simulink model "IEEE33BusTestSystemSimple"  (Simulink 10.3)
settings: Solver=FixedStepAuto  StartTime=0.0  StopTime=0.2  RelTol=1e-3
undefined symbols (not defined in the file): D1, Delta
libraries: spsThreePhaseVIMeasurementLib x43, spsThreePhaseSeriesRLCBranchLib x39, spsThreePhaseSeriesRLCLoadLib x34, simulink_extras x9, spsFrequencyPhasorLib x9, spsPowerPositiveSequenceLib x9, spsSequenceAnalyzerLib x9, spsThreePhaseParallelRLCLoadLib x3, spsSeriesRLCBranchLib x3, spsAC1AExcitationSystemLib x2, spsDieselMotorModel x2, spsSynchronousMachinepuStandardLib x2
(part 2 of 3)

== system IEEE33BusTestSystemSimple/Bus_18 ==
  Bus Load 18 : spsThreePhaseSeriesRLCLoadLib/Three-Phase Series RLC Load  LConnTagsString=A|B|C  Configuration=Y (grounded)  NominalVoltage=(12660)*0.91322  Vabc=[1e3 1e3 1e3]  Vabcp=[1e3 1e3 1e3]  NominalFrequency=50  UnbalancedPower=off  ActivePower=90e3  InductivePower=40e3  CapacitivePower=0  Pabc=[10e3 9e3 11e3]  QLabc=[100 90 110]  QCabc=[100 90 110]  Pabcp=[10e3 9e3 11e3]  QLabcp=[100 90 110]  QCabcp=[100 90 110]  Measurements=None  LoadType=constant PQ
  Bus_18 : spsThreePhaseVIMeasurementLib/Three-Phase V-I Measurement  VoltageMeasurement=phase-to-phase  SetLabelV=off  LabelV=Vabc  Vpu=off  VpuLL=off  CurrentMeasurement=yes  SetLabelI=off  LabelI=Iabc  Ipu=off  Pbase=100e6  Vbase=500e3  OutputType=Complex  PhasorSimulation=off  PSBequivalent=0
  VI Recorder21 : Subsystem
  InPhaseA : PMIOPort  Side=Left
  InPhaseB : PMIOPort  Port=2  Side=Left
  InPhaseC : PMIOPort  Port=3  Side=Left
  OutPhaseA : PMIOPort  Port=4  Side=Right
  OutPhaseB : PMIOPort  Port=5  Side=Right
  OutPhaseC : PMIOPort  Port=6  Side=Right
  wires:
  Bus_18/1 -> VI Recorder21/1(Vrec)
  Bus_18/2 -> VI Recorder21/2(Irec)
  connections:
  Bus Load 18/LConn1 -- OutPhaseA/RConn1 -- Bus_18/RConn1
  Bus_18/RConn2 -- OutPhaseB/RConn1 -- Bus Load 18/LConn2
  Bus_18/RConn3 -- OutPhaseC/RConn1 -- Bus Load 18/LConn3
  InPhaseA/RConn1 -- Bus_18/LConn1
  InPhaseB/RConn1 -- Bus_18/LConn2
  InPhaseC/RConn1 -- Bus_18/LConn3

== system IEEE33BusTestSystemSimple/Bus_19 ==
  Bus Load 19 : spsThreePhaseSeriesRLCLoadLib/Three-Phase Series RLC Load  LConnTagsString=A|B|C  Configuration=Y (grounded)  NominalVoltage=(12660)*0.996507  Vabc=[1e3 1e3 1e3]  Vabcp=[1e3 1e3 1e3]  NominalFrequency=50  UnbalancedPower=off  ActivePower=90e3  InductivePower=40e3  CapacitivePower=0  Pabc=[10e3 9e3 11e3]  QLabc=[100 90 110]  QCabc=[100 90 110]  Pabcp=[10e3 9e3 11e3]  QLabcp=[100 90 110]  QCabcp=[100 90 110]  Measurements=None  LoadType=constant PQ
  Bus_19 : spsThreePhaseVIMeasurementLib/Three-Phase V-I Measurement  VoltageMeasurement=phase-to-phase  SetLabelV=off  LabelV=Vabc  Vpu=off  VpuLL=off  CurrentMeasurement=yes  SetLabelI=off  LabelI=Iabc  Ipu=off  Pbase=100e6  Vbase=500e3  OutputType=Complex  PhasorSimulation=off  PSBequivalent=0
  VI Recorder : Subsystem
  InPhaseA : PMIOPort  Side=Left
  InPhaseB : PMIOPort  Port=2  Side=Left
  InPhaseC : PMIOPort  Port=3  Side=Left
  OutPhaseA : PMIOPort  Port=4  Side=Right
  OutPhaseB : PMIOPort  Port=5  Side=Right
  OutPhaseC : PMIOPort  Port=6  Side=Right
  wires:
  Bus_19/2 -> VI Recorder/2(Irec)
  Bus_19/1 -> VI Recorder/1(Vrec)
  connections:
  Bus Load 19/LConn1 -- OutPhaseA/RConn1 -- Bus_19/RConn1
  Bus_19/RConn2 -- OutPhaseB/RConn1 -- Bus Load 19/LConn2
  Bus Load 19/LConn3 -- OutPhaseC/RConn1 -- Bus_19/RConn3
  Bus_19/LConn1 -- InPhaseA/RConn1
  InPhaseB/RConn1 -- Bus_19/LConn2
  InPhaseC/RConn1 -- Bus_19/LConn3

== system IEEE33BusTestSystemSimple/Bus_2 ==
  Bus Load 2 : spsThreePhaseSeriesRLCLoadLib/Three-Phase Series RLC Load  LConnTagsString=A|B|C  Configuration=Y (grounded)  NominalVoltage=(12660)*0.997035  Vabc=[1e3 1e3 1e3]  Vabcp=[1e3 1e3 1e3]  NominalFrequency=50  UnbalancedPower=off  ActivePower=100e3  InductivePower=60e3  CapacitivePower=0  Pabc=[10e3 9e3 11e3]  QLabc=[100 90 110]  QCabc=[100 90 110]  Pabcp=[10e3 9e3 11e3]  QLabcp=[100 90 110]  QCabcp=[100 90 110]  Measurements=None  LoadType=constant PQ
  Bus_2 : spsThreePhaseVIMeasurementLib/Three-Phase V-I Measurement  VoltageMeasurement=phase-to-phase  SetLabelV=off  LabelV=Vabc  Vpu=off  VpuLL=off  CurrentMeasurement=yes  SetLabelI=off  LabelI=Iabc  Ipu=off  Pbase=100e6  Vbase=500e3  OutputType=Complex  PhasorSimulation=off  PSBequivalent=0
  VI Recorder5 : Subsystem
  InPhaseA : PMIOPort  Side=Left
  InPhaseB : PMIOPort  Port=2  Side=Left
  InPhaseC : PMIOPort  Port=3  Side=Left
  OutPhaseA1 : PMIOPort  Port=4  Side=Right
  OutPhaseB1 : PMIOPort  Port=5  Side=Right
  OutPhaseC1 : PMIOPort  Port=6  Side=Right
  OutPhaseA : PMIOPort  Port=7  Side=Right
  OutPhaseB : PMIOPort  Port=8  Side=Right
  OutPhaseC : PMIOPort  Port=9  Side=Right
  wires:
  Bus_2/2 -> VI Recorder5/2(Irec)
  Bus_2/1 -> VI Recorder5/1(Vrec)
  connections:
  InPhaseC/RConn1 -- Bus_2/LConn3
  InPhaseB/RConn1 -- Bus_2/LConn2
  InPhaseA/RConn1 -- Bus_2/LConn1
  Bus Load 2/LConn1 -- OutPhaseA1/RConn1 -- OutPhaseA/RConn1 -- Bus_2/RConn1
  Bus Load 2/LConn2 -- OutPhaseB1/RConn1 -- OutPhaseB/RConn1 -- Bus_2/RConn2
  Bus Load 2/LConn3 -- OutPhaseC1/RConn1 -- OutPhaseC/RConn1 -- Bus_2/RConn3

== system IEEE33BusTestSystemSimple/Bus_20 ==
  Bus Load 20 : spsThreePhaseSeriesRLCLoadLib/Three-Phase Series RLC Load  LConnTagsString=A|B|C  Configuration=Y (grounded)  NominalVoltage=(12660)*0.992929  Vabc=[1e3 1e3 1e3]  Vabcp=[1e3 1e3 1e3]  NominalFrequency=50  UnbalancedPower=off  ActivePower=90e3  InductivePower=40e3  CapacitivePower=0  Pabc=[10e3 9e3 11e3]  QLabc=[100 90 110]  QCabc=[100 90 110]  Pabcp=[10e3 9e3 11e3]  QLabcp=[100 90 110]  QCabcp=[100 90 110]  Measurements=None  LoadType=constant PQ
  Bus_20 : spsThreePhaseVIMeasurementLib/Three-Phase V-I Measurement  VoltageMeasurement=phase-to-phase  SetLabelV=off  LabelV=Vabc  Vpu=off  VpuLL=off  CurrentMeasurement=yes  SetLabelI=off  LabelI=Iabc  Ipu=off  Pbase=100e6  Vbase=500e3  OutputType=Complex  PhasorSimulation=off  PSBequivalent=0
  VI Recorder1 : Subsystem
  InPhaseA : PMIOPort  Side=Left
  InPhaseB : PMIOPort  Port=2  Side=Left
  InPhaseC : PMIOPort  Port=3  Side=Left
  OutPhaseA : PMIOPort  Port=4  Side=Right
  OutPhaseB : PMIOPort  Port=5  Side=Right
  OutPhaseC : PMIOPort  Port=6  Side=Right
  wires:
  Bus_20/1 -> VI Recorder1/1(Vrec)
  Bus_20/2 -> VI Recorder1/2(Irec)
  connections:
  Bus Load 20/LConn1 -- OutPhaseA/RConn1 -- Bus_20/RConn1
  Bus_20/RConn2 -- OutPhaseB/RConn1 -- Bus Load 20/LConn2
  Bus Load 20/LConn3 -- OutPhaseC/RConn1 -- Bus_20/RConn3
  InPhaseA/RConn1 -- Bus_20/LConn1
  InPhaseB/RConn1 -- Bus_20/LConn2
  InPhaseC/RConn1 -- Bus_20/LConn3

== system IEEE33BusTestSystemSimple/Bus_21 ==
  Bus Load 21 : spsThreePhaseSeriesRLCLoadLib/Three-Phase Series RLC Load  LConnTagsString=A|B|C  Configuration=Y (grounded)  NominalVoltage=(12660)*0.992224  Vabc=[1e3 1e3 1e3]  Vabcp=[1e3 1e3 1e3]  NominalFrequency=50  UnbalancedPower=off  ActivePower=90e3  InductivePower=40e3  CapacitivePower=0  Pabc=[10e3 9e3 11e3]  QLabc=[100 90 110]  QCabc=[100 90 110]  Pabcp=[10e3 9e3 11e3]  QLabcp=[100 90 110]  QCabcp=[100 90 110]  Measurements=None  LoadType=constant PQ
  Bus_21 : spsThreePhaseVIMeasurementLib/Three-Phase V-I Measurement  VoltageMeasurement=phase-to-phase  SetLabelV=off  LabelV=Vabc  Vpu=off  VpuLL=off  CurrentMeasurement=yes  SetLabelI=off  LabelI=Iabc  Ipu=off  Pbase=100e6  Vbase=500e3  OutputType=Complex  PhasorSimulation=off  PSBequivalent=0
  VI Recorder2 : Subsystem
  InPhaseA : PMIOPort  Side=Left
  InPhaseB : PMIOPort  Port=2  Side=Left
  InPhaseC : PMIOPort  Port=3  Side=Left
  OutPhaseA : PMIOPort  Port=4  Side=Right
  OutPhaseB : PMIOPort  Port=5  Side=Right
  OutPhaseC : PMIOPort  Port=6  Side=Right
  OutPhaseA1 : PMIOPort  Port=7  Side=Right
  OutPhaseB1 : PMIOPort  Port=8  Side=Right
  OutPhaseC1 : PMIOPort  Port=9  Side=Right
  wires:
  Bus_21/2 -> VI Recorder2/2(Irec)
  Bus_21/1 -> VI Recorder2/1(Vrec)
  connections:
  Bus_21/RConn1 -- OutPhaseA/RConn1 -- OutPhaseA1/RConn1 -- Bus Load 21/LConn1
  Bus_21/RConn2 -- OutPhaseB/RConn1 -- OutPhaseB1/RConn1 -- Bus Load 21/LConn2
  InPhaseA/RConn1 -- Bus_21/LConn1
  Bus_21/LConn2 -- InPhaseB/RConn1
  InPhaseC/RConn1 -- Bus_21/LConn3
  Bus Load 21/LConn3 -- OutPhaseC/RConn1 -- OutPhaseC1/RConn1 -- Bus_21/RConn3

== system IEEE33BusTestSystemSimple/Bus_22 ==
  Bus Load 22 : spsThreePhaseSeriesRLCLoadLib/Three-Phase Series RLC Load  LConnTagsString=A|B|C  Configuration=Y (grounded)  NominalVoltage=(12660)*0.991587  Vabc=[1e3 1e3 1e3]  Vabcp=[1e3 1e3 1e3]  NominalFrequency=50  UnbalancedPower=off  ActivePower=90e3  InductivePower=40e3  CapacitivePower=0  Pabc=[10e3 9e3 11e3]  QLabc=[100 90 110]  QCabc=[100 90 110]  Pabcp=[10e3 9e3 11e3]  QLabcp=[100 90 110]  QCabcp=[100 90 110]  Measurements=None  LoadType=constant PQ
  Bus_22 : spsThreePhaseVIMeasurementLib/Three-Phase V-I Measurement  VoltageMeasurement=phase-to-phase  SetLabelV=off  LabelV=Vabc  Vpu=off  VpuLL=off  CurrentMeasurement=yes  SetLabelI=off  LabelI=Iabc  Ipu=off  Pbase=100e6  Vbase=500e3  OutputType=Complex  PhasorSimulation=off  PSBequivalent=0
  VI Recorder3 : Subsystem
  InPhaseA : PMIOPort  Side=Left
  InPhaseB : PMIOPort  Port=2  Side=Left
  InPhaseC : PMIOPort  Port=3  Side=Left
  OutPhaseA : PMIOPort  Port=4  Side=Right
  OutPhaseB : PMIOPort  Port=5  Side=Right
  OutPhaseC : PMIOPort  Port=6  Side=Right
  wires:
  Bus_22/2 -> VI Recorder3/2(Irec)
  Bus_22/1 -> VI Recorder3/1(Vrec)
  connections:
  Bus_22/RConn2 -- OutPhaseB/RConn1 -- Bus Load 22/LConn2
  Bus Load 22/LConn3 -- OutPhaseC/RConn1 -- Bus_22/RConn3
  Bus_22/RConn1 -- OutPhaseA/RConn1 -- Bus Load 22/LConn1
  InPhaseA/RConn1 -- Bus_22/LConn1
  InPhaseB/RConn1 -- Bus_22/LConn2
  InPhaseC/RConn1 -- Bus_22/LConn3

== system IEEE33BusTestSystemSimple/Bus_23 ==
  Bus Load 23 : spsThreePhaseSeriesRLCLoadLib/Three-Phase Series RLC Load  LConnTagsString=A|B|C  Configuration=Y (grounded)  NominalVoltage=(12660)*0.97937  Vabc=[1e3 1e3 1e3]  Vabcp=[1e3 1e3 1e3]  NominalFrequency=50  UnbalancedPower=off  ActivePower=90e3  InductivePower=50e3  CapacitivePower=0  Pabc=[10e3 9e3 11e3]  QLabc=[100 90 110]  QCabc=[100 90 110]  Pabcp=[10e3 9e3 11e3]  QLabcp=[100 90 110]  QCabcp=[100 90 110]  Measurements=None  LoadType=constant PQ
  Bus_23 : spsThreePhaseVIMeasurementLib/Three-Phase V-I Measurement  VoltageMeasurement=phase-to-phase  SetLabelV=off  LabelV=Vabc  Vpu=off  VpuLL=off  CurrentMeasurement=yes  SetLabelI=off  LabelI=Iabc  Ipu=off  Pbase=100e6  Vbase=500e3  OutputType=Complex  PhasorSimulation=off  PSBequivalent=0
  VI Recorder32 : Subsystem
  InPhaseA : PMIOPort  Side=Left
  InPhaseB : PMIOPort  Port=2  Side=Left
  InPhaseC : PMIOPort  Port=3  Side=Left
  OutPhaseA : PMIOPort  Port=4  Side=Right
  OutPhaseB : PMIOPort  Port=5  Side=Right
  OutPhaseC : PMIOPort  Port=6  Side=Right
  wires:
  Bus_23/2 -> VI Recorder32/2(Irec)
  Bus_23/1 -> VI Recorder32/1(Vrec)
  connections:
  Bus Load 23/LConn1 -- OutPhaseA/RConn1 -- Bus_23/RConn1
  Bus_23/RConn2 -- OutPhaseB/RConn1 -- Bus Load 23/LConn2
  Bus_23/RConn3 -- OutPhaseC/RConn1 -- Bus Load 23/LConn3
  InPhaseA/RConn1 -- Bus_23/LConn1
  InPhaseB/RConn1 -- Bus_23/LConn2
  InPhaseC/RConn1 -- Bus_23/LConn3

== system IEEE33BusTestSystemSimple/Bus_24 ==
  Bus Load 24 : spsThreePhaseSeriesRLCLoadLib/Three-Phase Series RLC Load  LConnTagsString=A|B|C  Configuration=Y (grounded)  NominalVoltage=(12660)*0.9727  Vabc=[1e3 1e3 1e3]  Vabcp=[1e3 1e3 1e3]  NominalFrequency=50  UnbalancedPower=off  ActivePower=420e3  InductivePower=200e3  CapacitivePower=0  Pabc=[10e3 9e3 11e3]  QLabc=[100 90 110]  QCabc=[100 90 110]  Pabcp=[10e3 9e3 11e3]  QLabcp=[100 90 110]  QCabcp=[100 90 110]  Measurements=None  LoadType=constant PQ
  Bus_24 : spsThreePhaseVIMeasurementLib/Three-Phase V-I Measurement  VoltageMeasurement=phase-to-phase  SetLabelV=off  LabelV=Vabc  Vpu=off  VpuLL=off  CurrentMeasurement=yes  SetLabelI=off  LabelI=Iabc  Ipu=off  Pbase=100e6  Vbase=500e3  OutputType=Complex  PhasorSimulation=off  PSBequivalent=0
  VI Recorder31 : Subsystem
  InPhaseA : PMIOPort  Side=Left
  InPhaseB : PMIOPort  Port=2  Side=Left
  InPhaseC : PMIOPort  Port=3  Side=Left
  OutPhaseA : PMIOPort  Port=4  Side=Right
  OutPhaseB : PMIOPort  Port=5  Side=Right
  OutPhaseC : PMIOPort  Port=6  Side=Right
  wires:
  Bus_24/1 -> VI Recorder31/1(Vrec)
  Bus_24/2 -> VI Recorder31/2(Irec)
  connections:
  Bus Load 24/LConn1 -- Bus_24/RConn1 -- OutPhaseA/RConn1
  Bus_24/RConn2 -- OutPhaseB/RConn1 -- Bus Load 24/LConn2
  Bus_24/RConn3 -- OutPhaseC/RConn1 -- Bus Load 24/LConn3
  InPhaseA/RConn1 -- Bus_24/LConn1
  InPhaseB/RConn1 -- Bus_24/LConn2
  InPhaseC/RConn1 -- Bus_24/LConn3

== system IEEE33BusTestSystemSimple/Bus_25 ==
  Bus Load 25 : spsThreePhaseSeriesRLCLoadLib/Three-Phase Series RLC Load  LConnTagsString=A|B|C  Configuration=Y (grounded)  NominalVoltage=(12660)*0.969375  Vabc=[1e3 1e3 1e3]  Vabcp=[1e3 1e3 1e3]  NominalFrequency=50  UnbalancedPower=off  ActivePower=420e3  InductivePower=200e3  CapacitivePower=0  Pabc=[10e3 9e3 11e3]  QLabc=[100 90 110]  QCabc=[100 90 110]  Pabcp=[10e3 9e3 11e3]  QLabcp=[100 90 110]  QCabcp=[100 90 110]  Measurements=None  LoadType=constant PQ
  Bus_25 : spsThreePhaseVIMeasurementLib/Three-Phase V-I Measurement  VoltageMeasurement=phase-to-phase  SetLabelV=off  LabelV=Vabc  Vpu=off  VpuLL=off  CurrentMeasurement=yes  SetLabelI=off  LabelI=Iabc  Ipu=off  Pbase=100e6  Vbase=500e3  OutputType=Complex  PhasorSimulation=off  PSBequivalent=0
  VI Recorder30 : Subsystem
  InPhaseA : PMIOPort  Side=Left
  InPhaseB : PMIOPort  Port=2  Side=Left
  InPhaseC : PMIOPort  Port=3  Side=Left
  OutPhaseA : PMIOPort  Port=4  Side=Right
  OutPhaseB : PMIOPort  Port=5  Side=Right
  OutPhaseC : PMIOPort  Port=6  Side=Right
  wires:
  Bus_25/2 -> VI Recorder30/2(Irec)
  Bus_25/1 -> VI Recorder30/1(Vrec)
  connections:
  Bus Load 25/LConn1 -- OutPhaseA/RConn1 -- Bus_25/RConn1
  Bus_25/RConn2 -- OutPhaseB/RConn1 -- Bus Load 25/LConn2
  Bus Load 25/LConn3 -- OutPhaseC/RConn1 -- Bus_25/RConn3
  InPhaseB/RConn1 -- Bus_25/LConn2
  InPhaseA/RConn1 -- Bus_25/LConn1
  InPhaseC/RConn1 -- Bus_25/LConn3

== system IEEE33BusTestSystemSimple/Bus_26 ==
  Bus Load 26 : spsThreePhaseSeriesRLCLoadLib/Three-Phase Series RLC Load  LConnTagsString=A|B|C  Configuration=Y (grounded)  NominalVoltage=(12660)*0.947798  Vabc=[1e3 1e3 1e3]  Vabcp=[1e3 1e3 1e3]  NominalFrequency=50  UnbalancedPower=off  ActivePower=60e3  InductivePower=25e3  CapacitivePower=0  Pabc=[10e3 9e3 11e3]  QLabc=[100 90 110]  QCabc=[100 90 110]  Pabcp=[10e3 9e3 11e3]  QLabcp=[100 90 110]  QCabcp=[100 90 110]  Measurements=None  LoadType=constant PQ
  Bus_26 : spsThreePhaseVIMeasurementLib/Three-Phase V-I Measurement  VoltageMeasurement=phase-to-phase  SetLabelV=off  LabelV=Vabc  Vpu=off  VpuLL=off  CurrentMeasurement=yes  SetLabelI=off  LabelI=Iabc  Ipu=off  Pbase=100e6  Vbase=500e3  OutputType=Complex  PhasorSimulation=off  PSBequivalent=0
  VI Recorder22 : Subsystem
  InPhaseA : PMIOPort  Side=Left
  InPhaseB : PMIOPort  Port=2  Side=Left
  InPhaseC : PMIOPort  Port=3  Side=Left
  OutPhaseA : PMIOPort  Port=4  Side=Right
  OutPhaseB : PMIOPort  Port=5  Side=Right
  OutPhaseC : PMIOPort  Port=6  Side=Right
  wires:
  Bus_26/2 -> VI Recorder22/2(Irec)
  Bus_26/1 -> VI Recorder22/1(Vrec)
  connections:
  Bus_26/RConn2 -- OutPhaseB/RConn1 -- Bus Load 26/LConn2
  Bus Load 26/LConn3 -- OutPhaseC/RConn1 -- Bus_26/RConn3
  Bus Load 26/LConn1 -- OutPhaseA/RConn1 -- Bus_26/RConn1
  InPhaseA/RConn1 -- Bus_26/LConn1
  InPhaseB/RConn1 -- Bus_26/LConn2
  InPhaseC/RConn1 -- Bus_26/LConn3

== system IEEE33BusTestSystemSimple/Bus_27 ==
  Bus Load 27 : spsThreePhaseSeriesRLCLoadLib/Three-Phase Series RLC Load  LConnTagsString=A|B|C  Configuration=Y (grounded)  NominalVoltage=(12660)*0.945238  Vabc=[1e3 1e3 1e3]  Vabcp=[1e3 1e3 1e3]  NominalFrequency=50  UnbalancedPower=off  ActivePower=60e3  InductivePower=25e3  CapacitivePower=0  Pabc=[10e3 9e3 11e3]  QLabc=[100 90 110]  QCabc=[100 90 110]  Pabcp=[10e3 9e3 11e3]  QLabcp=[100 90 110]  QCabcp=[100 90 110]  Measurements=None  LoadType=constant PQ
  Bus_27 : spsThreePhaseVIMeasurementLib/Three-Phase V-I Measurement  VoltageMeasurement=phase-to-phase  SetLabelV=off  LabelV=Vabc  Vpu=off  VpuLL=off  CurrentMeasurement=yes  SetLabelI=off  LabelI=Iabc  Ipu=off  Pbase=100e6  Vbase=500e3  OutputType=Complex  PhasorSimulation=off  PSBequivalent=0
  VI Recorder23 : Subsystem
  InPhaseA : PMIOPort  Side=Left
  InPhaseB : PMIOPort  Port=2  Side=Left
  InPhaseC : PMIOPort  Port=3  Side=Left
  OutPhaseA : PMIOPort  Port=4  Side=Right
  OutPhaseB : PMIOPort  Port=5  Side=Right
  OutPhaseC : PMIOPort  Port=6  Side=Right
  wires:
  Bus_27/1 -> VI Recorder23/1(Vrec)
  Bus_27/2 -> VI Recorder23/2(Irec)
  connections:
  Bus_27/RConn1 -- OutPhaseA/RConn1 -- Bus Load 27/LConn1
  Bus_27/RConn2 -- OutPhaseB/RConn1 -- Bus Load 27/LConn2
  Bus Load 27/LConn3 -- OutPhaseC/RConn1 -- Bus_27/RConn3
  InPhaseA/RConn1 -- Bus_27/LConn1
  InPhaseB/RConn1 -- Bus_27/LConn2
  InPhaseC/RConn1 -- Bus_27/LConn3

== system IEEE33BusTestSystemSimple/Bus_28 ==
  Bus Load 28 : spsThreePhaseSeriesRLCLoadLib/Three-Phase Series RLC Load  LConnTagsString=A|B|C  Configuration=Y (grounded)  NominalVoltage=(12660)*0.933818  Vabc=[1e3 1e3 1e3]  Vabcp=[1e3 1e3 1e3]  NominalFrequency=50  UnbalancedPower=off  ActivePower=60e3  InductivePower=20e3  CapacitivePower=0  Pabc=[10e3 9e3 11e3]  QLabc=[100 90 110]  QCabc=[100 90 110]  Pabcp=[10e3 9e3 11e3]  QLabcp=[100 90 110]  QCabcp=[100 90 110]  Measurements=None  LoadType=constant PQ
  Bus_28 : spsThreePhaseVIMeasurementLib/Three-Phase V-I Measurement  VoltageMeasurement=phase-to-phase  SetLabelV=off  LabelV=Vabc  Vpu=off  VpuLL=off  CurrentMeasurement=yes  SetLabelI=off  LabelI=Iabc  Ipu=off  Pbase=100e6  Vbase=500e3  OutputType=Complex  PhasorSimulation=off  PSBequivalent=0
  VI Recorder24 : Subsystem
  InPhaseA : PMIOPort  Side=Left
  InPhaseB : PMIOPort  Port=2  Side=Left
  InPhaseC : PMIOPort  Port=3  Side=Left
  OutPhaseA : PMIOPort  Port=4  Side=Right
  OutPhaseB : PMIOPort  Port=5  Side=Right
  OutPhaseC : PMIOPort  Port=6  Side=Right
  wires:
  Bus_28/2 -> VI Recorder24/2(Irec)
  Bus_28/1 -> VI Recorder24/1(Vrec)
  connections:
  Bus_28/RConn1 -- OutPhaseA/RConn1 -- Bus Load 28/LConn1
  Bus_28/RConn2 -- OutPhaseB/RConn1 -- Bus Load 28/LConn2
  Bus_28/RConn3 -- OutPhaseC/RConn1 -- Bus Load 28/LConn3
  InPhaseA/RConn1 -- Bus_28/LConn1
  InPhaseB/RConn1 -- Bus_28/LConn2
  InPhaseC/RConn1 -- Bus_28/LConn3

== system IEEE33BusTestSystemSimple/Bus_29 ==
  Bus Load 29 : spsThreePhaseSeriesRLCLoadLib/Three-Phase Series RLC Load  LConnTagsString=A|B|C  Configuration=Y (grounded)  NominalVoltage=(12660)*0.925614  Vabc=[1e3 1e3 1e3]  Vabcp=[1e3 1e3 1e3]  NominalFrequency=50  UnbalancedPower=off  ActivePower=120e3  InductivePower=70e3  CapacitivePower=0  Pabc=[10e3 9e3 11e3]  QLabc=[100 90 110]  QCabc=[100 90 110]  Pabcp=[10e3 9e3 11e3]  QLabcp=[100 90 110]  QCabcp=[100 90 110]  Measurements=None  LoadType=constant PQ
  Bus_29 : spsThreePhaseVIMeasurementLib/Three-Phase V-I Measurement  VoltageMeasurement=phase-to-phase  SetLabelV=off  LabelV=Vabc  Vpu=off  VpuLL=off  CurrentMeasurement=yes  SetLabelI=off  LabelI=Iabc  Ipu=off  Pbase=100e6  Vbase=500e3  OutputType=Complex  PhasorSimulation=off  PSBequivalent=0
  VI Recorder25 : Subsystem
  InPhaseA : PMIOPort  Side=Left
  InPhaseB : PMIOPort  Port=2  Side=Left
  InPhaseC : PMIOPort  Port=3  Side=Left
  OutPhaseA : PMIOPort  Port=4  Side=Right
  OutPhaseB : PMIOPort  Port=5  Side=Right
  OutPhaseC : PMIOPort  Port=6  Side=Right
  InPhaseA1 : PMIOPort  Port=7  Side=Left
  InPhaseB1 : PMIOPort  Port=8  Side=Left
  InPhaseC1 : PMIOPort  Port=9  Side=Left
  wires:
  Bus_29/1 -> VI Recorder25/1(Vrec)
  Bus_29/2 -> VI Recorder25/2(Irec)
  connections:
  Bus Load 29/LConn1 -- OutPhaseA/RConn1 -- Bus_29/RConn1
  Bus_29/RConn2 -- OutPhaseB/RConn1 -- Bus Load 29/LConn2
  Bus_29/RConn3 -- OutPhaseC/RConn1 -- Bus Load 29/LConn3
  InPhaseB1/RConn1 -- InPhaseB/RConn1 -- Bus_29/LConn2
  InPhaseA1/RConn1 -- InPhaseA/RConn1 -- Bus_29/LConn1
  InPhaseC1/RConn1 -- InPhaseC/RConn1 -- Bus_29/LConn3

== system IEEE33BusTestSystemSimple/Bus_3 ==
  Bus Load 3 : spsThreePhaseSeriesRLCLoadLib/Three-Phase Series RLC Load  LConnTagsString=A|B|C  Configuration=Y (grounded)  NominalVoltage=(12660)*0.982955  Vabc=[1e3 1e3 1e3]  Vabcp=[1e3 1e3 1e3]  NominalFrequency=50  UnbalancedPower=off  ActivePower=90e3  InductivePower=40e3  CapacitivePower=0  Pabc=[10e3 9e3 11e3]  QLabc=[100 90 110]  QCabc=[100 90 110]  Pabcp=[10e3 9e3 11e3]  QLabcp=[100 90 110]  QCabcp=[100 90 110]  Measurements=None  LoadType=constant PQ
  Bus_3 : spsThreePhaseVIMeasurementLib/Three-Phase V-I Measurement  VoltageMeasurement=phase-to-phase  SetLabelV=off  LabelV=Vabc  Vpu=off  VpuLL=off  CurrentMeasurement=yes  SetLabelI=off  LabelI=Iabc  Ipu=off  Pbase=100e6  Vbase=500e3  OutputType=Complex  PhasorSimulation=off  PSBequivalent=0
  VI Recorder6 : Subsystem
  InPhaseA : PMIOPort  Side=Left
  InPhaseB : PMIOPort  Port=2  Side=Left
  InPhaseC : PMIOPort  Port=3  Side=Left
  OutPhaseA : PMIOPort  Port=4  Side=Right
  OutPhaseB : PMIOPort  Port=5  Side=Right
  OutPhaseC : PMIOPort  Port=6  Side=Right
  OutPhaseA1 : PMIOPort  Port=7  Side=Right
  OutPhaseB1 : PMIOPort  Port=8  Side=Right
  OutPhaseC1 : PMIOPort  Port=9  Side=Right
  wires:
  Bus_3/2 -> VI Recorder6/2(Irec)
  Bus_3/1 -> VI Recorder6/1(Vrec)
  connections:
  Bus Load 3/LConn1 -- OutPhaseA/RConn1 -- OutPhaseA1/RConn1 -- Bus_3/RConn1
  Bus_3/RConn2 -- OutPhaseB/RConn1 -- OutPhaseB1/RConn1 -- Bus Load 3/LConn2
  Bus Load 3/LConn3 -- OutPhaseC/RConn1 -- OutPhaseC1/RConn1 -- Bus_3/RConn3
  InPhaseA/RConn1 -- Bus_3/LConn1
  InPhaseB/RConn1 -- Bus_3/LConn2
  InPhaseC/RConn1 -- Bus_3/LConn3

== system IEEE33BusTestSystemSimple/Bus_30 ==
  Bus Load 30 : spsThreePhaseSeriesRLCLoadLib/Three-Phase Series RLC Load  LConnTagsString=A|B|C  Configuration=Y (grounded)  NominalVoltage=(12660)*0.922063  Vabc=[1e3 1e3 1e3]  Vabcp=[1e3 1e3 1e3]  NominalFrequency=50  UnbalancedPower=off  ActivePower=200e3  InductivePower=600e3  CapacitivePower=0  Pabc=[10e3 9e3 11e3]  QLabc=[100 90 110]  QCabc=[100 90 110]  Pabcp=[10e3 9e3 11e3]  QLabcp=[100 90 110]  QCabcp=[100 90 110]  Measurements=None  LoadType=constant PQ
  Bus_30 : spsThreePhaseVIMeasurementLib/Three-Phase V-I Measurement  VoltageMeasurement=phase-to-phase  SetLabelV=off  LabelV=Vabc  Vpu=off  VpuLL=off  CurrentMeasurement=yes  SetLabelI=off  LabelI=Iabc  Ipu=off  Pbase=100e6  Vbase=500e3  OutputType=Complex  PhasorSimulation=off  PSBequivalent=0
  VI Recorder26 : Subsystem
  InPhaseA : PMIOPort  Side=Left
  InPhaseB : PMIOPort  Port=2  Side=Left
  InPhaseC : PMIOPort  Port=3  Side=Left
  OutPhaseA : PMIOPort  Port=4  Side=Right
  OutPhaseB : PMIOPort  Port=5  Side=Right
  OutPhaseC : PMIOPort  Port=6  Side=Right
  wires:
  Bus_30/1 -> VI Recorder26/1(Vrec)
  Bus_30/2 -> VI Recorder26/2(Irec)
  connections:
  Bus Load 30/LConn1 -- OutPhaseA/RConn1 -- Bus_30/RConn1
  Bus_30/RConn2 -- OutPhaseB/RConn1 -- Bus Load 30/LConn2
  Bus_30/RConn3 -- OutPhaseC/RConn1 -- Bus Load 30/LConn3
  InPhaseB/RConn1 -- Bus_30/LConn2
  InPhaseA/RConn1 -- Bus_30/LConn1
  InPhaseC/RConn1 -- Bus_30/LConn3

== system IEEE33BusTestSystemSimple/Bus_31 ==
  Bus Load 31 : spsThreePhaseSeriesRLCLoadLib/Three-Phase Series RLC Load  LConnTagsString=A|B|C  Configuration=Y (grounded)  NominalVoltage=(12660)*0.917909  Vabc=[1e3 1e3 1e3]  Vabcp=[1e3 1e3 1e3]  NominalFrequency=50  UnbalancedPower=off  ActivePower=150e3  InductivePower=70e3  CapacitivePower=0  Pabc=[10e3 9e3 11e3]  QLabc=[100 90 110]  QCabc=[100 90 110]  Pabcp=[10e3 9e3 11e3]  QLabcp=[100 90 110]  QCabcp=[100 90 110]  Measurements=None  LoadType=constant PQ
  Bus_31 : spsThreePhaseVIMeasurementLib/Three-Phase V-I Measurement  VoltageMeasurement=phase-to-phase  SetLabelV=off  LabelV=Vabc  Vpu=off  VpuLL=off  CurrentMeasurement=yes  SetLabelI=off  LabelI=Iabc  Ipu=off  Pbase=100e6  Vbase=500e3  OutputType=Complex  PhasorSimulation=off  PSBequivalent=0
  VI Recorder27 : Subsystem
  InPhaseA : PMIOPort  Side=Left
  InPhaseB : PMIOPort  Port=2  Side=Left
  InPhaseC : PMIOPort  Port=3  Side=Left
  OutPhaseA : PMIOPort  Port=4  Side=Right
  OutPhaseB : PMIOPort  Port=5  Side=Right
  OutPhaseC : PMIOPort  Port=6  Side=Right
  wires:
  Bus_31/2 -> VI Recorder27/2(Irec)
  Bus_31/1 -> VI Recorder27/1(Vrec)
  connections:
  Bus Load 31/LConn1 -- OutPhaseA/RConn1 -- Bus_31/RConn1
  Bus_31/RConn2 -- OutPhaseB/RConn1 -- Bus Load 31/LConn2
  Bus_31/RConn3 -- OutPhaseC/RConn1 -- Bus Load 31/LConn3
  InPhaseA/RConn1 -- Bus_31/LConn1
  Bus_31/LConn2 -- InPhaseB/RConn1
  InPhaseC/RConn1 -- Bus_31/LConn3

== system IEEE33BusTestSystemSimple/Bus_32 ==
  Bus Load 32 : spsThreePhaseSeriesRLCLoadLib/Three-Phase Series RLC Load  LConnTagsString=A|B|C  Configuration=Y (grounded)  NominalVoltage=(12660)*0.916995  Vabc=[1e3 1e3 1e3]  Vabcp=[1e3 1e3 1e3]  NominalFrequency=50  UnbalancedPower=off  ActivePower=210e3  InductivePower=100e3  CapacitivePower=0  Pabc=[10e3 9e3 11e3]  QLabc=[100 90 110]  QCabc=[100 90 110]  Pabcp=[10e3 9e3 11e3]  QLabcp=[100 90 110]  QCabcp=[100 90 110]  Measurements=None  LoadType=constant PQ
  Bus_32 : spsThreePhaseVIMeasurementLib/Three-Phase V-I Measurement  VoltageMeasurement=phase-to-phase  SetLabelV=off  LabelV=Vabc  Vpu=off  VpuLL=off  CurrentMeasurement=yes  SetLabelI=off  LabelI=Iabc  Ipu=off  Pbase=100e6  Vbase=500e3  OutputType=Complex  PhasorSimulation=off  PSBequivalent=0
  VI Recorder28 : Subsystem
  InPhaseA : PMIOPort  Side=Left
  InPhaseB : PMIOPort  Port=2  Side=Left
  InPhaseC : PMIOPort  Port=3  Side=Left
  OutPhaseA : PMIOPort  Port=4  Side=Right
  OutPhaseB : PMIOPort  Port=5  Side=Right
  OutPhaseC : PMIOPort  Port=6  Side=Right
  wires:
  Bus_32/2 -> VI Recorder28/2(Irec)
  Bus_32/1 -> VI Recorder28/1(Vrec)
  connections:
  Bus Load 32/LConn1 -- OutPhaseA/RConn1 -- Bus_32/RConn1
  Bus_32/RConn2 -- OutPhaseB/RConn1 -- Bus Load 32/LConn2
  Bus Load 32/LConn3 -- OutPhaseC/RConn1 -- Bus_32/RConn3
  InPhaseA/RConn1 -- Bus_32/LConn1
  InPhaseB/RConn1 -- Bus_32/LConn2
  InPhaseC/RConn1 -- Bus_32/LConn3

== system IEEE33BusTestSystemSimple/Bus_33 ==
  Bus Load 33 : spsThreePhaseSeriesRLCLoadLib/Three-Phase Series RLC Load  LConnTagsString=A|B|C  Configuration=Y (grounded)  NominalVoltage=(12660)*0.916712  Vabc=[1e3 1e3 1e3]  Vabcp=[1e3 1e3 1e3]  NominalFrequency=50  UnbalancedPower=off  ActivePower=60e3  InductivePower=40e3  CapacitivePower=0  Pabc=[10e3 9e3 11e3]  QLabc=[100 90 110]  QCabc=[100 90 110]  Pabcp=[10e3 9e3 11e3]  QLabcp=[100 90 110]  QCabcp=[100 90 110]  Measurements=None  LoadType=constant PQ
  Bus_33 : spsThreePhaseVIMeasurementLib/Three-Phase V-I Measurement  VoltageMeasurement=phase-to-phase  SetLabelV=off  LabelV=Vabc  Vpu=off  VpuLL=off  CurrentMeasurement=yes  SetLabelI=off  LabelI=Iabc  Ipu=off  Pbase=100e6  Vbase=500e3  OutputType=Complex  PhasorSimulation=off  PSBequivalent=0
  VI Recorder29 : Subsystem
  InPhaseA : PMIOPort  Side=Left
  InPhaseB : PMIOPort  Port=2  Side=Left
  InPhaseC : PMIOPort  Port=3  Side=Left
  OutPhaseA : PMIOPort  Port=4  Side=Right
  OutPhaseB : PMIOPort  Port=5  Side=Right
  OutPhaseC : PMIOPort  Port=6  Side=Right
  wires:
  Bus_33/2 -> VI Recorder29/2(Irec)
  Bus_33/1 -> VI Recorder29/1(Vrec)
  connections:
  Bus Load 33/LConn1 -- Bus_33/RConn1 -- OutPhaseA/RConn1
  Bus Load 33/LConn2 -- OutPhaseB/RConn1 -- Bus_33/RConn2
  Bus_33/RConn3 -- OutPhaseC/RConn1 -- Bus Load 33/LConn3
  InPhaseA/RConn1 -- Bus_33/LConn1
  InPhaseB/RConn1 -- Bus_33/LConn2
  InPhaseC/RConn1 -- Bus_33/LConn3

== system IEEE33BusTestSystemSimple/Bus_4 ==
  Bus Load 4 : spsThreePhaseSeriesRLCLoadLib/Three-Phase Series RLC Load  LConnTagsString=A|B|C  Configuration=Y (grounded)  NominalVoltage=(12660)*0.975484  Vabc=[1e3 1e3 1e3]  Vabcp=[1e3 1e3 1e3]  NominalFrequency=50  UnbalancedPower=off  ActivePower=120e3  InductivePower=80e3  CapacitivePower=0  Pabc=[10e3 9e3 11e3]  QLabc=[100 90 110]  QCabc=[100 90 110]  Pabcp=[10e3 9e3 11e3]  QLabcp=[100 90 110]  QCabcp=[100 90 110]  Measurements=None  LoadType=constant PQ
  Bus_4 : spsThreePhaseVIMeasurementLib/Three-Phase V-I Measurement  VoltageMeasurement=phase-to-phase  SetLabelV=off  LabelV=Vabc  Vpu=off  VpuLL=off  CurrentMeasurement=yes  SetLabelI=off  LabelI=Iabc  Ipu=off  Pbase=100e6  Vbase=500e3  OutputType=Complex  PhasorSimulation=off  PSBequivalent=0
  VI Recorder7 : Subsystem
  InPhaseA : PMIOPort  Side=Left
  InPhaseB : PMIOPort  Port=2  Side=Left
  InPhaseC : PMIOPort  Port=3  Side=Left
  OutPhaseA : PMIOPort  Port=4  Side=Right
  OutPhaseB : PMIOPort  Port=5  Side=Right
  OutPhaseC : PMIOPort  Port=6  Side=Right
  wires:
  Bus_4/1 -> VI Recorder7/1(Vrec)
  Bus_4/2 -> VI Recorder7/2(Irec)
  connections:
  Bus Load 4/LConn1 -- OutPhaseA/RConn1 -- Bus_4/RConn1
  Bus_4/RConn2 -- OutPhaseB/RConn1 -- Bus Load 4/LConn2
  Bus Load 4/LConn3 -- OutPhaseC/RConn1 -- Bus_4/RConn3
  InPhaseA/RConn1 -- Bus_4/LConn1
  InPhaseB/RConn1 -- Bus_4/LConn2
  InPhaseC/RConn1 -- Bus_4/LConn3

== system IEEE33BusTestSystemSimple/Bus_5 ==
  Bus Load 5 : spsThreePhaseSeriesRLCLoadLib/Three-Phase Series RLC Load  LConnTagsString=A|B|C  Configuration=Y (grounded)  NominalVoltage=(12660)*0.968098  Vabc=[1e3 1e3 1e3]  Vabcp=[1e3 1e3 1e3]  NominalFrequency=50  UnbalancedPower=off  ActivePower=60e3  InductivePower=30e3  CapacitivePower=0  Pabc=[10e3 9e3 11e3]  QLabc=[100 90 110]  QCabc=[100 90 110]  Pabcp=[10e3 9e3 11e3]  QLabcp=[100 90 110]  QCabcp=[100 90 110]  Measurements=None  LoadType=constant PQ
  Bus_5 : spsThreePhaseVIMeasurementLib/Three-Phase V-I Measurement  VoltageMeasurement=phase-to-phase  SetLabelV=off  LabelV=Vabc  Vpu=off  VpuLL=off  CurrentMeasurement=yes  SetLabelI=off  LabelI=Iabc  Ipu=off  Pbase=100e6  Vbase=500e3  OutputType=Complex  PhasorSimulation=off  PSBequivalent=0
  VI Recorder8 : Subsystem
  InPhaseA : PMIOPort  Side=Left
  InPhaseB : PMIOPort  Port=2  Side=Left
  InPhaseC : PMIOPort  Port=3  Side=Left
  OutPhaseA : PMIOPort  Port=4  Side=Right
  OutPhaseB : PMIOPort  Port=5  Side=Right
  OutPhaseC : PMIOPort  Port=6  Side=Right
  wires:
  Bus_5/2 -> VI Recorder8/2(Irec)
  Bus_5/1 -> VI Recorder8/1(Vrec)
  connections:
  Bus_5/RConn1 -- OutPhaseA/RConn1 -- Bus Load 5/LConn1
  Bus Load 5/LConn2 -- OutPhaseB/RConn1 -- Bus_5/RConn2
  Bus Load 5/LConn3 -- OutPhaseC/RConn1 -- Bus_5/RConn3
  InPhaseA/RConn1 -- Bus_5/LConn1
  InPhaseB/RConn1 -- Bus_5/LConn2
  InPhaseC/RConn1 -- Bus_5/LConn3

== system IEEE33BusTestSystemSimple/Bus_6 ==
  Bus Load 6 : spsThreePhaseSeriesRLCLoadLib/Three-Phase Series RLC Load  LConnTagsString=A|B|C  Configuration=Y (grounded)  NominalVoltage=(12660)*0.949724  Vabc=[1e3 1e3 1e3]  Vabcp=[1e3 1e3 1e3]  NominalFrequency=50  UnbalancedPower=off  ActivePower=60e3  InductivePower=20e3  CapacitivePower=0  Pabc=[10e3 9e3 11e3]  QLabc=[100 90 110]  QCabc=[100 90 110]  Pabcp=[10e3 9e3 11e3]  QLabcp=[100 90 110]  QCabcp=[100 90 110]  Measurements=None  LoadType=constant PQ
  Bus_6 : spsThreePhaseVIMeasurementLib/Three-Phase V-I Measurement  VoltageMeasurement=phase-to-phase  SetLabelV=off  LabelV=Vabc  Vpu=off  VpuLL=off  CurrentMeasurement=yes  SetLabelI=off  LabelI=Iabc  Ipu=off  Pbase=100e6  Vbase=500e3  OutputType=Complex  PhasorSimulation=off  PSBequivalent=0
  VI Recorder9 : Subsystem
  InPhaseA : PMIOPort  Side=Left
  InPhaseB : PMIOPort  Port=2  Side=Left
  InPhaseC : PMIOPort  Port=3  Side=Left
  OutPhaseA : PMIOPort  Port=4  Side=Right
  OutPhaseB : PMIOPort  Port=5  Side=Right
  OutPhaseC : PMIOPort  Port=6  Side=Right
  OutPhaseA1 : PMIOPort  Port=7  Side=Right
  OutPhaseB1 : PMIOPort  Port=8  Side=Right
  OutPhaseC1 : PMIOPort  Port=9  Side=Right
  wires:
  Bus_6/1 -> VI Recorder9/1(Vrec)
  Bus_6/2 -> VI Recorder9/2(Irec)
  connections:
  Bus_6/RConn1 -- OutPhaseA/RConn1 -- OutPhaseA1/RConn1 -- Bus Load 6/LConn1
  Bus_6/RConn2 -- OutPhaseB/RConn1 -- OutPhaseB1/RConn1 -- Bus Load 6/LConn2
  Bus_6/RConn3 -- OutPhaseC/RConn1 -- OutPhaseC1/RConn1 -- Bus Load 6/LConn3
  InPhaseA/RConn1 -- Bus_6/LConn1
  InPhaseB/RConn1 -- Bus_6/LConn2
  InPhaseC/RConn1 -- Bus_6/LConn3

== system IEEE33BusTestSystemSimple/Bus_7 ==
  Bus Load 7 : spsThreePhaseSeriesRLCLoadLib/Three-Phase Series RLC Load  LConnTagsString=A|B|C  Configuration=Y (grounded)  NominalVoltage=(12660)*0.946243  Vabc=[1e3 1e3 1e3]  Vabcp=[1e3 1e3 1e3]  NominalFrequency=50  UnbalancedPower=off  ActivePower=200e3  InductivePower=100e3  CapacitivePower=0  Pabc=[10e3 9e3 11e3]  QLabc=[100 90 110]  QCabc=[100 90 110]  Pabcp=[10e3 9e3 11e3]  QLabcp=[100 90 110]  QCabcp=[100 90 110]  Measurements=None  LoadType=constant PQ
  Bus_7 : spsThreePhaseVIMeasurementLib/Three-Phase V-I Measurement  VoltageMeasurement=phase-to-phase  SetLabelV=off  LabelV=Vabc  Vpu=off  VpuLL=off  CurrentMeasurement=yes  SetLabelI=off  LabelI=Iabc  Ipu=off  Pbase=100e6  Vbase=500e3  OutputType=Complex  PhasorSimulation=off  PSBequivalent=0
  VI Recorder10 : Subsystem
  InPhaseA : PMIOPort  Side=Left
  InPhaseB : PMIOPort  Port=2  Side=Left
  InPhaseC : PMIOPort  Port=3  Side=Left
  OutPhaseA : PMIOPort  Port=4  Side=Right
  OutPhaseB : PMIOPort  Port=5  Side=Right
  OutPhaseC : PMIOPort  Port=6  Side=Right
  wires:
  Bus_7/2 -> VI Recorder10/2(Irec)
  Bus_7/1 -> VI Recorder10/1(Vrec)
  connections:
  Bus Load 7/LConn1 -- OutPhaseA/RConn1 -- Bus_7/RConn1
  Bus_7/RConn2 -- OutPhaseB/RConn1 -- Bus Load 7/LConn2
  InPhaseA/RConn1 -- Bus_7/LConn1
  InPhaseB/RConn1 -- Bus_7/LConn2
  InPhaseC/RConn1 -- Bus_7/LConn3
  OutPhaseC/RConn1 -- Bus Load 7/LConn3 -- Bus_7/RConn3

== system IEEE33BusTestSystemSimple/Bus_8 ==
  Bus Load 8 : spsThreePhaseSeriesRLCLoadLib/Three-Phase Series RLC Load  LConnTagsString=A|B|C  Configuration=Y (grounded)  NominalVoltage=(12660)*0.941407  Vabc=[1e3 1e3 1e3]  Vabcp=[1e3 1e3 1e3]  NominalFrequency=50  UnbalancedPower=off  ActivePower=200e3  InductivePower=100e3  CapacitivePower=0  Pabc=[10e3 9e3 11e3]  QLabc=[100 90 110]  QCabc=[100 90 110]  Pabcp=[10e3 9e3 11e3]  QLabcp=[100 90 110]  QCabcp=[100 90 110]  Measurements=None  LoadType=constant PQ
  Bus_8 : spsThreePhaseVIMeasurementLib/Three-Phase V-I Measurement  VoltageMeasurement=phase-to-phase  SetLabelV=off  LabelV=Vabc  Vpu=off  VpuLL=off  CurrentMeasurement=yes  SetLabelI=off  LabelI=Iabc  Ipu=off  Pbase=100e6  Vbase=500e3  OutputType=Complex  PhasorSimulation=off  PSBequivalent=0
  VI Recorder11 : Subsystem
  InPhaseA : PMIOPort  Side=Left
  InPhaseB : PMIOPort  Port=2  Side=Left
  InPhaseC : PMIOPort  Port=3  Side=Left
  OutPhaseA : PMIOPort  Port=4  Side=Right
  OutPhaseB : PMIOPort  Port=5  Side=Right
  OutPhaseC : PMIOPort  Port=6  Side=Right
  InPhaseA1 : PMIOPort  Port=7  Side=Left
  InPhaseB1 : PMIOPort  Port=8  Side=Left
  InPhaseC1 : PMIOPort  Port=9  Side=Left
  wires:
  Bus_8/2 -> VI Recorder11/2(Irec)
  Bus_8/1 -> VI Recorder11/1(Vrec)
  connections:
  Bus_8/RConn1 -- OutPhaseA/RConn1 -- Bus Load 8/LConn1
  Bus_8/RConn2 -- OutPhaseB/RConn1 -- Bus Load 8/LConn2
  Bus Load 8/LConn3 -- OutPhaseC/RConn1 -- Bus_8/RConn3
  InPhaseA1/RConn1 -- InPhaseA/RConn1 -- Bus_8/LConn1
  InPhaseB1/RConn1 -- InPhaseB/RConn1 -- Bus_8/LConn2
  InPhaseC1/RConn1 -- InPhaseC/RConn1 -- Bus_8/LConn3

== system IEEE33BusTestSystemSimple/Bus_9 ==
  Bus Load 9 : spsThreePhaseSeriesRLCLoadLib/Three-Phase Series RLC Load  LConnTagsString=A|B|C  Configuration=Y (grounded)  NominalVoltage=(12660)*0.935148  Vabc=[1e3 1e3 1e3]  Vabcp=[1e3 1e3 1e3]  NominalFrequency=50  UnbalancedPower=off  ActivePower=60e3  InductivePower=20e3  CapacitivePower=0  Pabc=[10e3 9e3 11e3]  QLabc=[100 90 110]  QCabc=[100 90 110]  Pabcp=[10e3 9e3 11e3]  QLabcp=[100 90 110]  QCabcp=[100 90 110]  Measurements=None  LoadType=constant PQ
  Bus_9 : spsThreePhaseVIMeasurementLib/Three-Phase V-I Measurement  VoltageMeasurement=phase-to-phase  SetLabelV=off  LabelV=Vabc  Vpu=off  VpuLL=off  CurrentMeasurement=yes  SetLabelI=off  LabelI=Iabc  Ipu=off  Pbase=100e6  Vbase=500e3  OutputType=Complex  PhasorSimulation=off  PSBequivalent=0
  VI Recorder12 : Subsystem
  InPhaseA : PMIOPort  Side=Left
  InPhaseB : PMIOPort  Port=2  Side=Left
  InPhaseC : PMIOPort  Port=3  Side=Left
  OutPhaseA : PMIOPort  Port=4  Side=Right
  OutPhaseB : PMIOPort  Port=5  Side=Right
  OutPhaseC : PMIOPort  Port=6  Side=Right
  OutPhaseA1 : PMIOPort  Port=7  Side=Right
  OutPhaseB1 : PMIOPort  Port=8  Side=Right
  OutPhaseC1 : PMIOPort  Port=9  Side=Right
  wires:
  Bus_9/2 -> VI Recorder12/2(Irec)
  Bus_9/1 -> VI Recorder12/1(Vrec)
  connections:
  Bus_9/RConn1 -- OutPhaseA/RConn1 -- OutPhaseA1/RConn1 -- Bus Load 9/LConn1
  Bus Load 9/LConn2 -- OutPhaseB/RConn1 -- OutPhaseB1/RConn1 -- Bus_9/RConn2
  Bus_9/RConn3 -- OutPhaseC/RConn1 -- OutPhaseC1/RConn1 -- Bus Load 9/LConn3
  InPhaseA/RConn1 -- Bus_9/LConn1
  InPhaseB/RConn1 -- Bus_9/LConn2
  InPhaseC/RConn1 -- Bus_9/LConn3

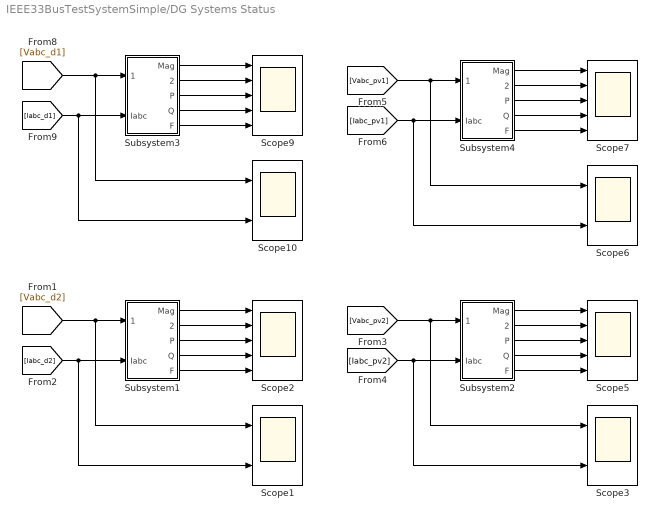
== system IEEE33BusTestSystemSimple/DG Systems Status ==
  Scope{1,3,6,10} (4 alike) : Scope  NumInputPorts=2
  Scope{2,5,7,9} (4 alike) : Scope  NumInputPorts=5
  Subsystem1 : Subsystem
  Subsystem2 : Subsystem
  Subsystem3 : Subsystem
  Subsystem4 : Subsystem
  wires:
  Subsystem1/3(P) -> Scope2/3
  [Vabc_pv1] -> Subsystem4/1(Vabc), Scope6/1
  Subsystem1/5(F) -> Scope2/5
  Subsystem4/2(Phase) -> Scope7/2
  Subsystem3/4(Q) -> Scope9/4
  Subsystem1/4(Q) -> Scope2/4
  Subsystem4/5(F) -> Scope7/5
  Subsystem2/1(Mag) -> Scope5/1
  Subsystem2/4(Q) -> Scope5/4
  Subsystem3/5(F) -> Scope9/5
  [Iabc_pv1] -> Subsystem4/2(Iabc), Scope6/2
  [Vabc_d2] -> Subsystem1/1(Vabc), Scope1/1
  [Vabc_d1] -> Subsystem3/1(Vabc), Scope10/1
  Subsystem2/2(Phase) -> Scope5/2
  [Iabc_d2] -> Subsystem1/2(Iabc), Scope1/2
  Subsystem3/3(P) -> Scope9/3
  Subsystem4/3(P) -> Scope7/3
  [Iabc_pv2] -> Subsystem2/2(Iabc), Scope3/2
  Subsystem4/4(Q) -> Scope7/4
  Subsystem4/1(Mag) -> Scope7/1
  Subsystem3/2(Phase) -> Scope9/2
  Subsystem1/2(Phase) -> Scope2/2
  Subsystem3/1(Mag) -> Scope9/1
  Subsystem1/1(Mag) -> Scope2/1
  [Iabc_d1] -> Subsystem3/2(Iabc), Scope10/2
  [Vabc_pv2] -> Subsystem2/1(Vabc), Scope3/1
  Subsystem2/3(P) -> Scope5/3
  Subsystem2/5(F) -> Scope5/5

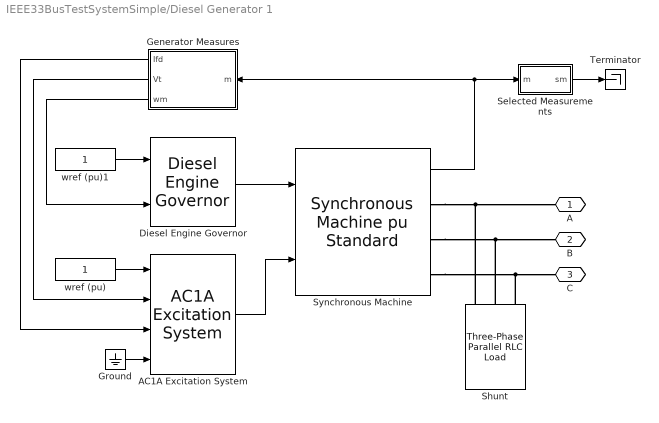
== system IEEE33BusTestSystemSimple/Diesel Generator 1 ==
  AC1A Excitation System : spsAC1AExcitationSystemLib/AC1A Excitation System  Tr=20e-3  KaTa=[400 0.02]  VAminmax=[-14.5 14.5]  VRminmax=[-5.43 6.03]  KfTf=[0.03 1.0]  TbTc=[0 0]  KeTe=[1.0 0.80]  Ve12=[4.18 3.14]  SeVe12=[0.10 0.03]  Kd=0.38  Kc=0.20  v0=[1.0064 1.0079]  TsBlock=0
      settings: SourceProductBaseCode=PS
  Diesel Engine Governor : spsDieselMotorModel/Diesel Engine Governor  K=29  Tr=[0.01 0.02 0.2]  Ta=[0.25 0.009 0.0384]  Tlim=[0 1.1]  Td=0.024  Pm0=0.050008
      settings: SourceProductBaseCode=PS
  Generator Measures : Subsystem
  Ground : Ground
  Selected Measurements : Subsystem
  Shunt : spsThreePhaseParallelRLCLoadLib/Three-Phase Parallel RLC Load  LConnTagsString=A|B|C  Configuration=Y (grounded)  NominalVoltage=12.66e3  Vabc=[1e3 1e3 1e3]  Vabcp=[1e3 1e3 1e3]  NominalFrequency=50  UnbalancedPower=off  ActivePower=0.05*2e6  InductivePower=0  CapacitivePower=0  Pabc=[10e3 9e3 11e3]  QLabc=[100 90 110]  QCabc=[100 90 110]  Pabcp=[10e3 9e3 11e3]  QLabcp=[100 90 110]  QCabcp=[100 90 110]  Measurements=None  LoadType=constant Z
  Synchronous Machine : spsSynchronousMachinepuStandardLib/Synchronous Machine pu Standard  PresetModel=No  MechanicalLoad=Mechanical power Pm  ShowDetailedParameters=on  RotorType=Salient-pole  Units=per unit standard parameters  MeasurementBus=off  NominalParameters=[ 2e6 12.66e3 50]  Reactances1=[ 1.81, 0.3, 0.23, 1.76, 0.65, 0.25, 0.15 ]  Reactances2="[ 1.305, 0.296, 0.252, 0.474,  0.243,  0.18 ]"  dAxisTimeConstants=Open-circuit  qAxisTimeConstants=Short-circuit  TimeConstants1="[ 4.4849  0.0681  0.1  ]"  TimeConstants2=[ 8.0, 0.03, 1.0, 0.07 ]  TimeConstants3="[  4.49  0.0681  0.0513  ]"  TimeConstants4=[ 8.0, 0.03, 0.3371, 0.0295 ]  TimeConstants5=[ 1.01, 0.053, 0.1 ]  TimeConstants6=[ 1.3201, 0.023, 1.0, 0.07 ]  TimeConstants7=[0.012 0.003 0.003]  TimeConstants8=[ 1.3201, 0.0231, 0.3371, 0.0295 ]  StatorResistance=0.003  Mechanical=[3.7 0 1 ]  PolePairs=20  InitialConditions=[0 -91.112 0.0485894 0.0387742 0.0672236 -23.7149 -103.71 121.673 1.00793]  SetSaturation=off  Saturation=[0.6404,0.7127,0.8441,0.9214,0.9956,1.082,1.19,1.316,1.457;0.7,0.7698,0.8872,0.9466,0.9969,1.046,1.1,1.151,1.201]  LoadFlowParameters=[1,0,0,0,0]  TsPowergui=0  TsBlock=-1  IterativeModel=Trapezoidal non iterative  IterativeDiscreteModel=Trapezoidal non iterative  BusType=PV  Pref=2e6  Qref=0  Qmin=-inf  Qmax=inf  PLF=0  QLF=0
      settings: SourceProductBaseCode=PS
  Terminator : Terminator
  wref (pu) : Constant
  wref (pu)1 : Constant
  A : PMIOPort  Side=Right
  B : PMIOPort  Port=2  Side=Right
  C : PMIOPort  Port=3  Side=Right
  wires:
  wref (pu)1/1 -> Diesel Engine Governor/1
  Diesel Engine Governor/1 -> Synchronous Machine/1
  AC1A Excitation System/1 -> Synchronous Machine/2
  wref (pu)/1 -> AC1A Excitation System/1
  Synchronous Machine/1 -> Generator Measures/1(m), Selected Measurements/1(m)
  Ground/1 -> AC1A Excitation System/4
  Generator Measures/3(wm) -> Diesel Engine Governor/2
  Generator Measures/2(Vt) -> AC1A Excitation System/2
  Generator Measures/1(Ifd) -> AC1A Excitation System/3
  Selected Measurements/1(sm) -> Terminator/1
  connections:
  Shunt/LConn1 -- Synchronous Machine/RConn1 -- A/RConn1
  Synchronous Machine/RConn3 -- Shunt/LConn3 -- C/RConn1
  Synchronous Machine/RConn2 -- Shunt/LConn2 -- B/RConn1

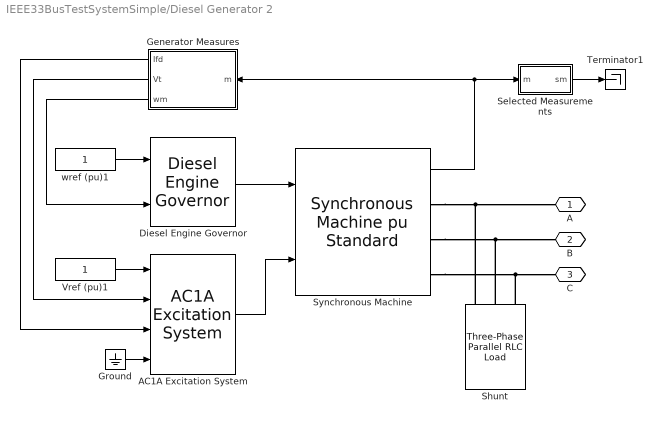
== system IEEE33BusTestSystemSimple/Diesel Generator 2 ==
  AC1A Excitation System : spsAC1AExcitationSystemLib/AC1A Excitation System  Tr=20e-3  KaTa=[400 0.02]  VAminmax=[-14.5 14.5]  VRminmax=[-5.43 6.03]  KfTf=[0.03 1.0]  TbTc=[0 0]  KeTe=[1.0 0.80]  Ve12=[4.18 3.14]  SeVe12=[0.10 0.03]  Kd=0.38  Kc=0.20  v0=[1.0064 1.0079]  TsBlock=0
      settings: SourceProductBaseCode=PS
  Diesel Engine Governor : spsDieselMotorModel/Diesel Engine Governor  K=29  Tr=[0.01 0.02 0.2]  Ta=[0.25 0.009 0.0384]  Tlim=[0 1.1]  Td=0.024  Pm0=0.050008
      settings: SourceProductBaseCode=PS
  Generator Measures : Subsystem
  Ground : Ground
  Selected Measurements : Subsystem
  Shunt : spsThreePhaseParallelRLCLoadLib/Three-Phase Parallel RLC Load  LConnTagsString=A|B|C  Configuration=Y (grounded)  NominalVoltage=12.66e3  Vabc=[1e3 1e3 1e3]  Vabcp=[1e3 1e3 1e3]  NominalFrequency=50  UnbalancedPower=off  ActivePower=0.05*1e6  InductivePower=0  CapacitivePower=0  Pabc=[10e3 9e3 11e3]  QLabc=[100 90 110]  QCabc=[100 90 110]  Pabcp=[10e3 9e3 11e3]  QLabcp=[100 90 110]  QCabcp=[100 90 110]  Measurements=None  LoadType=constant Z
  Synchronous Machine : spsSynchronousMachinepuStandardLib/Synchronous Machine pu Standard  PresetModel=No  MechanicalLoad=Mechanical power Pm  ShowDetailedParameters=on  RotorType=Salient-pole  Units=per unit standard parameters  MeasurementBus=off  NominalParameters=[ 1e6 12.66e3 50]  Reactances1=[ 1.81, 0.3, 0.23, 1.76, 0.65, 0.25, 0.15 ]  Reactances2="[ 1.305, 0.296, 0.252, 0.474,  0.243,  0.18 ]"  dAxisTimeConstants=Open-circuit  qAxisTimeConstants=Short-circuit  TimeConstants1="[ 4.4849  0.0681  0.1  ]"  TimeConstants2=[ 8.0, 0.03, 1.0, 0.07 ]  TimeConstants3="[  4.49  0.0681  0.0513  ]"  TimeConstants4=[ 8.0, 0.03, 0.3371, 0.0295 ]  TimeConstants5=[ 1.01, 0.053, 0.1 ]  TimeConstants6=[ 1.3201, 0.023, 1.0, 0.07 ]  TimeConstants7=[0.012 0.003 0.003]  TimeConstants8=[ 1.3201, 0.0231, 0.3371, 0.0295 ]  StatorResistance=0.003  Mechanical=[3.7 0 1 ]  PolePairs=20  InitialConditions=[0 -91.112 0.0485894 0.0387742 0.0672236 -23.7149 -103.71 121.673 1.00793]  SetSaturation=off  Saturation=[0.6404,0.7127,0.8441,0.9214,0.9956,1.082,1.19,1.316,1.457;0.7,0.7698,0.8872,0.9466,0.9969,1.046,1.1,1.151,1.201]  LoadFlowParameters=[1,0,0,0,0]  TsPowergui=0  TsBlock=-1  IterativeModel=Trapezoidal non iterative  IterativeDiscreteModel=Trapezoidal non iterative  BusType=PV  Pref=1e6  Qref=0  Qmin=-inf  Qmax=inf  PLF=0  QLF=0
      settings: SourceProductBaseCode=PS
  Terminator1 : Terminator
  Vref (pu)1 : Constant
  wref (pu)1 : Constant
  A : PMIOPort  Side=Right
  B : PMIOPort  Port=2  Side=Right
  C : PMIOPort  Port=3  Side=Right
  wires:
  wref (pu)1/1 -> Diesel Engine Governor/1
  Diesel Engine Governor/1 -> Synchronous Machine/1
  AC1A Excitation System/1 -> Synchronous Machine/2
  Vref (pu)1/1 -> AC1A Excitation System/1
  Synchronous Machine/1 -> Generator Measures/1(m), Selected Measurements/1(m)
  Ground/1 -> AC1A Excitation System/4
  Generator Measures/3(wm) -> Diesel Engine Governor/2
  Generator Measures/2(Vt) -> AC1A Excitation System/2
  Generator Measures/1(Ifd) -> AC1A Excitation System/3
  Selected Measurements/1(sm) -> Terminator1/1
  connections:
  Shunt/LConn1 -- Synchronous Machine/RConn1 -- A/RConn1
  Synchronous Machine/RConn3 -- Shunt/LConn3 -- C/RConn1
  Synchronous Machine/RConn2 -- Shunt/LConn2 -- B/RConn1

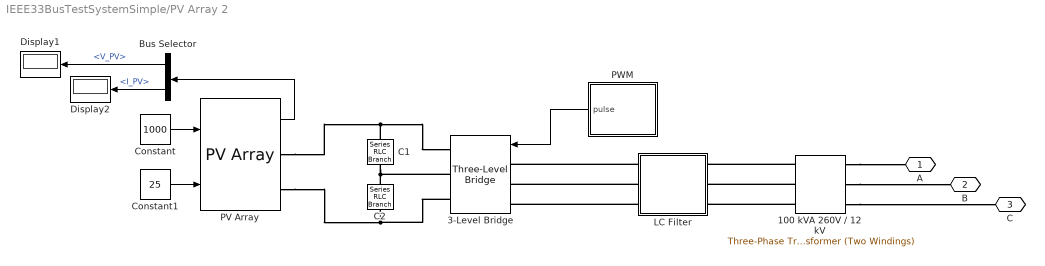
== system IEEE33BusTestSystemSimple/PV Array 2  ==
  100 kVA 260V / 12 kV : spsThreePhaseTransformerTwoWindingsLib/Three-Phase Transformer (Two Windings)  Winding1Connection=Yg  Winding2Connection=Delta (D1)  CoreType=Three single-phase transformers  SetSaturation=off  Hysteresis=off  DataFile='hysteresis'  SetInitialFlux=off  Measurements=None  UNITS=pu  NominalPower=[500e3 , 50 ]  Winding1=[ 12e3 , 0.001 , 0.03 ]  Winding2=[ 260 , 0.001 , 0.03 ]  Rm=500  Lm=500  L0=0.49999  Saturation=[ 0,0 ; 0.0024,1.2 ; 1.0,1.52 ]  InitialFluxes=[0.79999 -0.79999 0.70002]  BreakLoop=off  DiscreteSolver=Trapezoidal iterative  DataType=off  TransfoNumber=0
  3-Level Bridge : spsThreeLevelBridgeLib/Three-Level Bridge  Arms=3  SnubberResistance=1e6  SbubberCapacitance=inf  Device=IGBT / Diodes  Ron=0.2e-3  ForwardVoltages="[  0  0 ]"  Measurements=None
      settings: AttributesFormatString=\n  SourceProductBaseCode=PS
  Bus Selector : BusSelector  OutputSignals=V_PV,I_PV
  C1 : spsSeriesRLCBranchLib/Series RLC Branch  LConnTagsString=__new0  RConnTagsString=__new0  BranchType=C  Resistance=1.0  Inductance=1.0  SetiL0=off  InitialCurrent=0  Capacitance=12000e-06  Setx0=off  InitialVoltage=0  Measurements=None
  C2 : spsSeriesRLCBranchLib/Series RLC Branch  LConnTagsString=__new0  RConnTagsString=__new0  BranchType=C  Resistance=1.0  Inductance=1.0  SetiL0=off  InitialCurrent=0  Capacitance=12000e-06  Setx0=off  InitialVoltage=0  Measurements=None
  Constant : Constant  Value=1000
  Constant1 : Constant  Value=25
  Display1 : Display
  Display2 : Display
  LC Filter : Subsystem
  PV Array : spsPVArrayLib/PV Array  Npar=85  Nser=15  PlotType=array @ 1000 W/m2 & specified temperatures  S_vec="[ 1000  500  100 ]"  Temp_C_vec="[ 45 25  ]"  ModuleName=Sunpower SPR-E19-415-COM  PlotWhenSelected=off  Pm=414.801  Ncell=128  Voc=85.3  Isc=6.09  Vm=72.9  Im=5.69  beta_Voc_pc=-0.326  alpha_Isc_pc=0.018998  beta_Voc=-0.27808  alpha_Isc=0.001157  IL=6.0939  I0=5.5564e-11  nI=1.0214  Rsh=531.1106  Rs=0.33964  RobustModel=off  RobustCellTemperature=313.3991  BAL=off  Tc=1e-6  Tfilter=5e-5
  PWM : Subsystem
  A : PMIOPort  Side=Left
  B : PMIOPort  Port=2  Side=Left
  C : PMIOPort  Port=3  Side=Left
  wires:
  PV Array/1 -> Bus Selector/1
  Bus Selector/2 -> Display2/1  "<I_PV>"
  Bus Selector/1 -> Display1/1  "<V_PV>"
  Constant1/1 -> PV Array/2
  Constant/1 -> PV Array/1
  PWM/1(pulse) -> 3-Level Bridge/1
  connections:
  C1/LConn1 -- PV Array/RConn1 -- 3-Level Bridge/RConn1
  100 kVA 260V / 12 kV/LConn3 -- C/RConn1
  3-Level Bridge/RConn2 -- C1/RConn1 -- C2/LConn1
  3-Level Bridge/RConn3 -- PV Array/RConn2 -- C2/RConn1
  100 kVA 260V / 12 kV/LConn2 -- B/RConn1
  100 kVA 260V / 12 kV/LConn1 -- A/RConn1
  LC Filter/LConn1 -- 3-Level Bridge/LConn1
  100 kVA 260V / 12 kV/RConn1 -- LC Filter/RConn1
  LC Filter/LConn2 -- 3-Level Bridge/LConn2
  100 kVA 260V / 12 kV/RConn2 -- LC Filter/RConn2
  LC Filter/LConn3 -- 3-Level Bridge/LConn3
  100 kVA 260V / 12 kV/RConn3 -- LC Filter/RConn3

== system IEEE33BusTestSystemSimple/Solar Generator ==
  Bus Selector : BusSelector  OutputSignals=Active power P (W),Positive-sequence voltage V (pu),Reactive power Q (var)
  Constant11 : Constant  Value=0
  Mux1 : Mux  Inputs=2
  Scope5 : Scope  NumInputPorts=3
  Shunt : spsThreePhaseParallelRLCLoadLib/Three-Phase Parallel RLC Load  LConnTagsString=A|B|C  Configuration=Y (grounded)  NominalVoltage=12.66e3  Vabc=[1e3 1e3 1e3]  Vabcp=[1e3 1e3 1e3]  NominalFrequency=50  UnbalancedPower=off  ActivePower=0.05*1e6  InductivePower=0  CapacitivePower=0  Pabc=[10e3 9e3 11e3]  QLabc=[100 90 110]  QCabc=[100 90 110]  Pabcp=[10e3 9e3 11e3]  QLabcp=[100 90 110]  QCabcp=[100 90 110]  Measurements=None  LoadType=constant Z
  Simple Solar Inverter : spsThreePhaseDynamicLoadLib/Three-Phase Dynamic Load  NominalVoltage=[12.66e3 50]  ActiveReactivePowers=[-250000 -3.38813e-13]  PositiveSequence=[1.01061 -3.2037]  ExternalControl=on  NpNq=[1.3 2]  TimeConstants="[0  0  0  0]"  MinimumVoltage=0.7  Tfilter=1e-2  LoadFlowParameters=[4,0,0,0,0]
      settings: SourceProductBaseCode=PS
  Sine Wave : Sin  Amplitude=100e3  Bias=1e6  Frequency=0.05  SampleTime=0
  Unary Minus : UnaryMinus
  Unary Minus1 : UnaryMinus
  Unary Minus4 : UnaryMinus
  A : PMIOPort  Side=Right
  B : PMIOPort  Port=2  Side=Right
  C : PMIOPort  Port=3  Side=Right
  wires:
  Sine Wave/1 -> Unary Minus/1
  Unary Minus4/1 -> Scope5/3
  Bus Selector/2 -> Scope5/2  "<Positive-sequence voltage V (pu)>"
  Unary Minus/1 -> Mux1/1
  Mux1/1 -> Simple Solar Inverter/1
  Bus Selector/3 -> Unary Minus4/1  "<Reactive power Q (var)>"
  Unary Minus1/1 -> Scope5/1
  Bus Selector/1 -> Unary Minus1/1  "<Active power P (W)>"
  Constant11/1 -> Mux1/2
  Simple Solar Inverter/1 -> Bus Selector/1
  connections:
  Simple Solar Inverter/LConn1 -- Shunt/LConn1 -- A/RConn1
  Simple Solar Inverter/LConn2 -- Shunt/LConn2 -- B/RConn1
  Simple Solar Inverter/LConn3 -- C/RConn1 -- Shunt/LConn3
